simulink model "exp03e03_ped"  (Simulink 8.9)
settings: Solver=FixedStepAuto  StartTime=0.0  StopTime=1  FixedStep=0.0042  RelTol=1e-10  EnableMultiTasking=on
values from neighbouring files (symbols this model uses):
  c1 = 2.94    [prelab03.m]
  k1 = 338.6    [prelab03.m]
  kd = 0.01    [prelab03.m]
  khw = 14732    [prelab03.m]
  kp = 0.08    [prelab03.m]
  m1 = mc1 + mw1    (= 2.778)    [prelab03.m]
libraries: simulink_need_slupdate x1
settings Model: Creator=Giovani  LastModifiedBy=Gabriel
settings DataIOCC: LimitDataPoints=off
settings OptimizationCC: ExpressionDepthLimit=2147483647
settings DebuggingCC: SolverPrmCheckMsg=warning
settings GRTTargetCC: GeneratePreprocessorConditionals=Use local settings

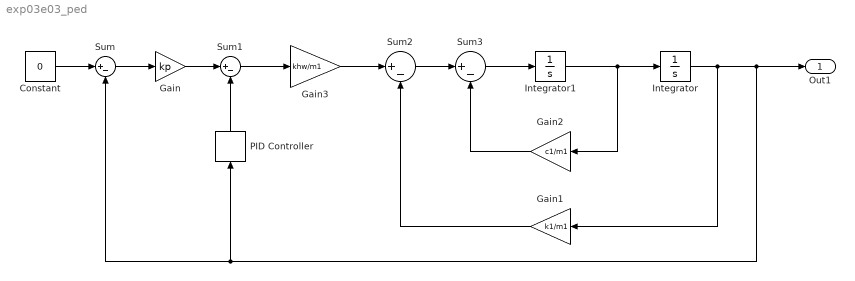
== system exp03e03_ped ==
  Constant : Constant  Value=0
  Gain : Gain  Gain=kp
  Gain1 : Gain  Gain=k1/m1
  Gain2 : Gain  Gain=c1/m1
  Gain3 : Gain  Gain=khw/m1
  Integrator : Integrator  InitialCondition=1000
  Integrator1 : Integrator
  PID Controller : simulink_need_slupdate/PID Controller  P=1  I=0  D=kd
      settings: SourceProductName=Simulink
  Sum{,1..3} (4 alike) : Sum  Inputs=|+-
  Out1 : Outport
  wires:
  Sum/1 -> Gain/1
  Gain/1 -> Sum1/1
  PID Controller/1 -> Sum1/2
  Sum3/1 -> Integrator1/1
  Gain1/1 -> Sum2/2
  Sum2/1 -> Sum3/1
  Integrator1/1 -> Integrator/1, Gain2/1
  Gain2/1 -> Sum3/2
  Gain3/1 -> Sum2/1
  Sum1/1 -> Gain3/1
  Integrator/1 -> Out1/1, Sum/2, PID Controller/1, Gain1/1
  Constant/1 -> Sum/1
